simulink model "questao6"  (R2021b)
settings: Solver=VariableStepAuto  StartTime=0.0  StopTime=1800  RelTol=1e-3
values from neighbouring files (symbols this model uses):
  A = [A11 A12 ... (first row only)    [main.m]
  B = [Bu Bd]    [main.m]
  C = [1 0]    [main.m]
  D = zeros(1,4)    [main.m]
  dF = 0    [main.m]
  dFj = 4.72e-5    (= 4.72e-05)    [main.m]
  dTi = 0    [main.m]
  dTij = 0    [main.m]
  ftd1 = c2d(ftc, 50)    [main.m]
  ftd2 = c2d(ftc, 150)    [main.m]
  ftd3 = c2d(ftc, 300)    [main.m]
  Ts = 51.67    [main.m]
settings Model: Creator=luang  LastModifiedBy=luang

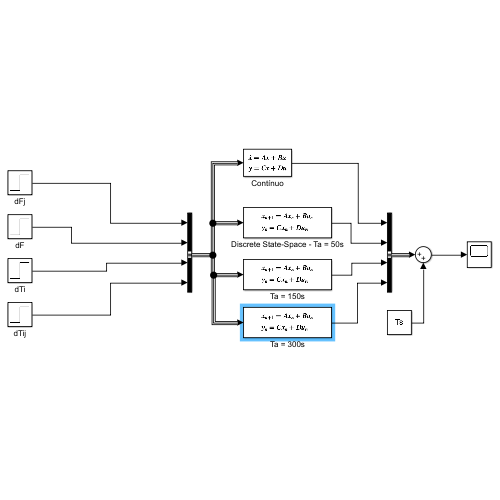
[thumbnail: Simulink's stored preview of the top-level diagram]
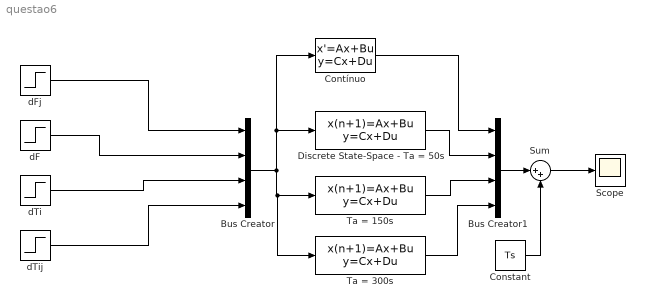
== system questao6 ==
  Bus Creator : BusCreator  Inputs=4
  Bus Creator1 : BusCreator  Inputs=4
  Constant : Constant  Value=Ts
  Contínuo : StateSpace  A=A  B=B  C=C  D=D  InitialCondition=0
  Discrete State-Space - Ta = 50s : DiscreteStateSpace  A=ftd1.A  B=ftd1.B  C=ftd1.C  D=ftd1.D  SampleTime=50
  Scope : Scope
  Sum : Sum  Inputs=|++
  Ta = 150s : DiscreteStateSpace  A=ftd2.A  B=ftd2.B  C=ftd2.C  D=ftd2.D  SampleTime=150
  Ta = 300s : DiscreteStateSpace  A=ftd3.A  B=ftd3.B  C=ftd3.C  D=ftd3.D  SampleTime=300
  dF : Step  After=dF  SampleTime=0
  dFj : Step  After=dFj  SampleTime=0
  dTi : Step  After=dTi  SampleTime=0
  dTij : Step  After=dTij  SampleTime=0
  wires:
  dTij/1 -> Bus Creator/4
  dFj/1 -> Bus Creator/1
  dF/1 -> Bus Creator/2
  dTi/1 -> Bus Creator/3
  Bus Creator/1 -> Ta = 300s/1, Ta = 150s/1, Discrete State-Space - Ta = 50s/1, Contínuo/1
  Contínuo/1 -> Bus Creator1/1
  Discrete State-Space - Ta = 50s/1 -> Bus Creator1/2
  Ta = 150s/1 -> Bus Creator1/3
  Ta = 300s/1 -> Bus Creator1/4
  Constant/1 -> Sum/2
  Bus Creator1/1 -> Sum/1
  Sum/1 -> Scope/1
